simulink model "v00_0A_0E"  (R2022b)
settings: Solver=FixedStepDiscrete  StartTime=0.0  StopTime=8000  FixedStep=SampleTime  MaxStep=Contactors_StepTime_msec  RelTol=1e-3  EnableMultiTasking=on
undefined symbols (not defined in the file): A_to_mA, BalancingTempGroup, canChannel, CapacityFactor, CC_Inputs, CellSOC, ChargeState, ContactorsFlags, DiscIntNeverNeededParam, gEN_Contactors_StepTime_msec, Ion, isDynamicCurrentEn, Lithium, maxAllowedImbalance, nCells_parallel, nCells_series, nCellTempGrps, PermanentFailRecoveryTrigger, ProtectionFlags, RBal_ohm, SampleTime, sigbuilder_block, StLineEq_varA, StLineEq_varB, TempSelectForDCL, Thresholds, V_to_mV
libraries: simulink x32, spsIdealSwitchLib x21, spsBatteryLib x20, spsSeriesRLCBranchLib x20, spsVoltageMeasurementLib x20, canmsglib x4, canlib x3, dspstat3 x2, spspowerguiLib x2, spsControlledCurrentSourceLib x1, spsCurrentMeasurementLib x1
(part 3 of 7)

== system v00_0A_0E/CellBalancing ==
  note: BalanceEn_atRest is added in Input Processing block for offline cell balancing
  note: BalanceEn = 1 is added in statemachine when transitioning from Lobby to even balancing
  BalancingTempGroup : Inport
  maxAllowedImbalance : Inport  Port=2
  StLineEq_varA : Inport  Port=3
  StLineEq_varB : Inport  Port=4
  Thresholds : Inport  Port=5
  DataPipeline : Inport  Port=6
  BalancingStateMachine : Stateflow chart  TreatAsAtomicUnit=on
      settings: PortSchema="{\"entries\":[{\"content\":{\"sides\":[{\"content\":{\"connectorIds\":[\"In1\",\"In3\",\"In2\",\"In4\",\"In6\",\"In5\"]},\"type\":\"ConnectorPlacement.EquallySpacedRectSide\",\"uuid\":\"2851f266-9e46-4eaf-8471-39569b09250f\"},{\"content\":{\"connectorIds\":[\"Out2\",\"Out1\"],\"side\":\"RIGHT\"},\"type\":\"ConnectorPlacement.EquallySpacedRectSide\",\"uuid\":\"62b89b69-68b5-43db-8812-bb8e11eec61f\"},{\"content\":{\"connectorIds\":[],\"side\":\"TOP\"},\"type\":\"ConnectorPlacement.EquallySpacedRectSide\",\"uuid\":\"40469b38-8e93-4311-b6ae-b85f5792b8b2\"},{\"content\":{\"connectorIds\":[],\"side\":\"BOTTOM\"},\"type\":\"ConnectorPlacement.EquallySpacedRectSide\",\"uuid\":\"8aed0a4d-23dc-44c4-b683-dda48b400f95\"}]},\"type\":\"ConnectorPlacement.EquallySpacedConnector\",\"uuid\":\"3b02c2cb-c692-4407-a922-660092207305\"}],\"packageUris\":[\"http://schema.mathworks.com/mf0/Connector/R2020b\"],\"version\":\"1.0\"}"
  Bus Creator : BusCreator  Inputs=3  OutDataTypeStr=Bus: CellBalancingOutputBus  NonVirtualBus=on
  Bus Selector1 : BusSelector  OutputSignals=VoltageSenseBus.mV_max,nCells_series,VoltageSenseBus.Voltages_mV,VoltageSenseBus.mV_min
  InputProcessing : Subsystem
  Subtract : Sum  Inputs=+-  AccumDataTypeStr=int32
  BalanceCmd : Outport
  CellBalancingOutput : Outport  Port=2
  wires:
  InputProcessing/1(BalanceEn) -> BalancingStateMachine/4(BalanceEn), Bus Creator/2  "BalanceEn"
  BalancingStateMachine/1(BalanceCmd) -> BalanceCmd/1  "BalanceCmd"
  DataPipeline/1 -> InputProcessing/1(DataPipeline), Bus Selector1/1  "DataPipeline"
  Thresholds/1 -> InputProcessing/6(Thresholds), BalancingStateMachine/5(Thresholds)  "Thresholds"
  Bus Creator/1 -> CellBalancingOutput/1  "CellBalancingOutput"
  StLineEq_varA/1 -> InputProcessing/3(StLineEq_varA)  "StLineEq_varA"
  StLineEq_varB/1 -> InputProcessing/4(StLineEq_varB)  "StLineEq_varB"
  BalancingTempGroup/1 -> InputProcessing/5(BalancingTempGroup)  "BalancingTempGroup"
  InputProcessing/2(BalancingTimeOn_msec) -> BalancingStateMachine/6(BalancingTimeOn_msec)  "BalancingTimeOn_msec"
  Bus Selector1/2 -> BalancingStateMachine/1(nCells_series)  "<nCells_series>"
  Bus Selector1/3 -> BalancingStateMachine/3(Voltage_mV)  "<Voltages_mV>"
  Subtract/1 -> Bus Creator/1  "MaxImbalance_mV"
  BalancingStateMachine/2(CurrentBalancingState) -> Bus Creator/3  "CurrentBalancingState"
  Bus Selector1/4 -> Subtract/2, BalancingStateMachine/2(mV_min)  "<mV_min>"
  Bus Selector1/1 -> Subtract/1  "<mV_max>"
  maxAllowedImbalance/1 -> InputProcessing/2(MaxAllowedImbalance)

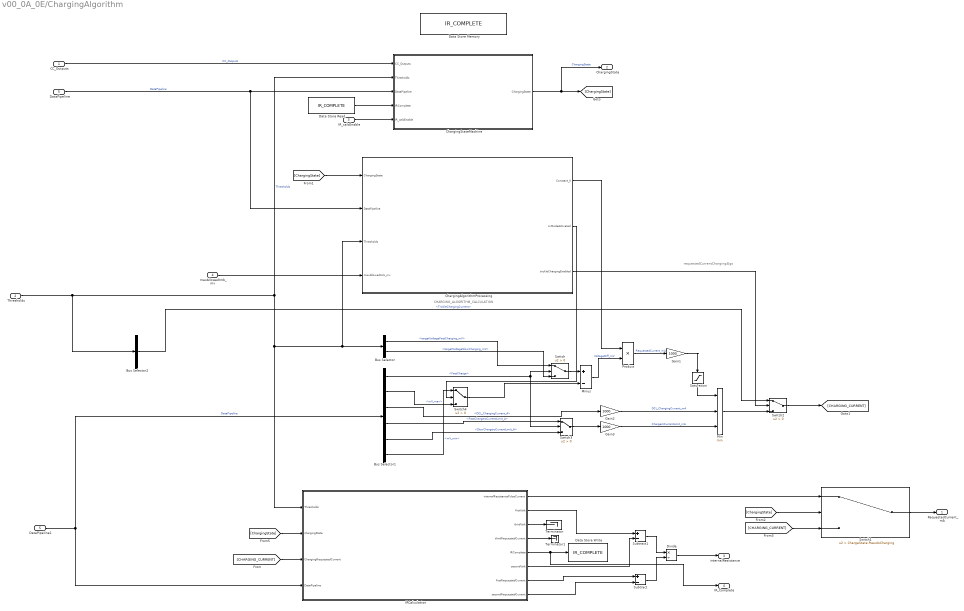
== system v00_0A_0E/ChargingAlgorithm ==
  note: requestedCurrentChargingAlgo
  note: CHARGING_ALGORITHM_CALCULATION
  CC_Outputs : Inport
  Thresholds : Inport  Port=2
  IR_calcEnable : Inport  Port=3
  maxAllowedImb_mv : Inport  Port=4
  DataPipeline : Inport  Port=5
  Bus Selector : BusSelector  OutputSignals=targetVoltageFastCharging_mV,targetVoltageSlowCharging_mV
  Bus Selector1 : BusSelector  OutputSignals=VCU.FastCharge,VoltageSenseBus.mV_max,DCL_ChargingCurrent_A,VCU.FastChargersCurrentLimit_A,VCU.SlowChargersCurrentLimit_A,VoltageSenseBus.mV_min
  Bus Selector2 : BusSelector  OutputSignals=TrickleChargingCurrent
  ChargingAlgorithmProcessing : Stateflow chart  TreatAsAtomicUnit=on
  ChargingStateMachine : Stateflow chart  TreatAsAtomicUnit=on
  Data Store Memory : DataStoreMemory  DataStoreName=IR_COMPLETE  WriteAfterWriteMsg=warning  ShowAdditionalParam=off  OutDataTypeStr=boolean
  Data Store Read : DataStoreRead  DataStoreName=IR_COMPLETE  IndexOptions=Index vector (dialog)  Indices=1  OutputSizes=1
  Data Store Write : DataStoreWrite  DataStoreName=IR_COMPLETE  IndexOptions=Index vector (dialog)  Indices=1  OutputSizes=1
  DataPipeline1 : InportShadow  Port=5
  Divide : Product  Inputs=*/  OutDataTypeStr=double
  Gain1 : Gain  Gain=1000
  Gain2 : Gain  Gain=1000
  Gain3 : Gain  Gain=1000
  IRCalculation : Stateflow chart  TreatAsAtomicUnit=on
      settings: PortSchema="{\"entries\":[{\"content\":{\"sides\":[{\"content\":{\"connectorIds\":[\"In3\",\"In2\",\"In4\",\"In1\"]},\"type\":\"ConnectorPlacement.EquallySpacedRectSide\",\"uuid\":\"09f3344b-a7a5-4c58-b859-bc86e5255ecc\"},{\"content\":{\"connectorIds\":[\"Out1\",\"Out5\",\"Out6\",\"Out7\",\"Out8\",\"Out4\",\"Out3\",\"Out2\"],\"side\":\"RIGHT\"},\"type\":\"ConnectorPlacement.EquallySpacedRectSide\",\"uuid\":\"d87cb124-6959-4bc9-a690-eca1c3acb93d\"},{\"content\":{\"connectorIds\":[],\"side\":\"TOP\"},\"type\":\"ConnectorPlacement.EquallySpacedRectSide\",\"uuid\":\"d4f2166d-1afb-4cd8-92f5-d7d1af5b4065\"}]},\"type\":\"ConnectorPlacement.EquallySpacedConnector\",\"uuid\":\"753fa2af-6988-4d89-a789-6b550e8286be\"}],\"packageUris\":[\"http://schema.mathworks.com/mf0/Connector/R2020b\"],\"version\":\"1.0\"}"
  Min : MinMax  Inputs=3
  Minus : Sum  Inputs=+-  OutDataTypeStr=int32
  Product : Product  OutDataTypeStr=int32
  Saturation : Saturate  UpperLimit=200000  LowerLimit=0
  Subtract : Sum  Inputs=+-
  Subtract1 : Sum  Inputs=+-
  Switch{,2..4} (4 alike) : Switch  Criteria=u2 > Threshold  SaturateOnIntegerOverflow=off  InputSameDT=off
  Switch1 : Switch  Criteria=u2 > Threshold  Threshold=ChargeState.PseudoCharging  SaturateOnIntegerOverflow=off  InputSameDT=off
  Terminator : Terminator
  Terminator1 : Terminator
  RequestedCurrent_mA : Outport
  ChargingState : Outport  Port=2
  internalResistance : Outport  Port=3
  IR_Complete : Outport  Port=4
  wires:
  IRCalculation/7(thirdRequestedCurrent) -> Terminator1/1
  IRCalculation/1(internalResistancePulseCurrent) -> Switch1/1
  Subtract/1 -> Divide/2
  IRCalculation/2(secondRequestedCurrent) -> Subtract/2
  IRCalculation/4(secondVolt) -> Subtract1/2
  IRCalculation/3(firstRequestedCurrent) -> Subtract/1
  IRCalculation/5(firstVolt) -> Subtract1/1
  Subtract1/1 -> Divide/1
  CC_Outputs/1 -> ChargingStateMachine/1(CC_Outputs)  "CC_Outputs"
  [ChargingState] -> ChargingAlgorithmProcessing/1(ChargingState)
  IRCalculation/6(thirdVolt) -> Terminator/1
  Bus Selector1/6 -> Switch4/1  "<mV_min>"
  Bus Selector2/1 -> Switch2/1  "<TrickleChargingCurrent>"
  Bus Selector1/3 -> Gain2/1  "<DCL_ChargingCurrent_A>"
  Gain3/1 -> Min/3  "ChargersCurrentLimit_mA"
  Bus Selector1/1 -> Switch3/2, Switch/2  "<FastCharge>"
  Switch3/1 -> Gain3/1
  Gain2/1 -> Min/2  "DCL_ChargingCurrent_mA"
  Minus/1 -> Product/2  "VoltageDiff_mV"
  ChargingAlgorithmProcessing/3(trickleChargingEnabled) -> Switch2/2
  Min/1 -> Switch2/3
  DataPipeline/1 -> ChargingAlgorithmProcessing/2(DataPipeline), ChargingStateMachine/3(DataPipeline)  "DataPipeline"
  Switch/1 -> Minus/1
  ChargingAlgorithmProcessing/1(Constant_K) -> Product/1
  DataPipeline1/1 -> Bus Selector1/1, IRCalculation/1(DataPipeline)  "DataPipeline"
  Product/1 -> Gain1/1  "RequestedCurrent_mA"
  Bus Selector1/5 -> Switch3/3  "<SlowChargersCurrentLimit_A>"
  ChargingAlgorithmProcessing/2(cvModeActivated) -> Switch4/2
  Bus Selector/2 -> Switch/3  "<targetVoltageSlowCharging_mV>"
  Thresholds/1 -> Bus Selector2/1, ChargingStateMachine/2(Thresholds), Bus Selector/1, ChargingAlgorithmProcessing/3(Thresholds), IRCalculation/3(Thresholds)  "Thresholds"
  Bus Selector1/4 -> Switch3/1  "<FastChargersCurrentLimit_A>"
  Bus Selector/1 -> Switch/1  "<targetVoltageFastCharging_mV>"
  Gain1/1 -> Saturation/1
  Switch4/1 -> Minus/2
  IR_calcEnable/1 -> ChargingStateMachine/5(IR_calcEnable)
  maxAllowedImb_mv/1 -> ChargingAlgorithmProcessing/4(maxAllowedImb_mv)
  Saturation/1 -> Min/1
  Bus Selector1/2 -> Switch4/3  "<mV_max>"
  [ChargingState] -> Switch1/2
  Switch1/1 -> RequestedCurrent_mA/1
  Switch2/1 -> [CHARGING_CURRENT]
  [CHARGING_CURRENT] -> IRCalculation/4(ChargingRequestedCurrent)
  [CHARGING_CURRENT] -> Switch1/3
  Divide/1 -> internalResistance/1
  IRCalculation/8(IRComplete) -> IR_Complete/1, Data Store Write/1
  Data Store Read/1 -> ChargingStateMachine/4(IRComplete)
  ChargingStateMachine/1(ChargingState) -> ChargingState/1, [ChargingState]  "ChargingState"
  [ChargingState] -> IRCalculation/2(chargingState)

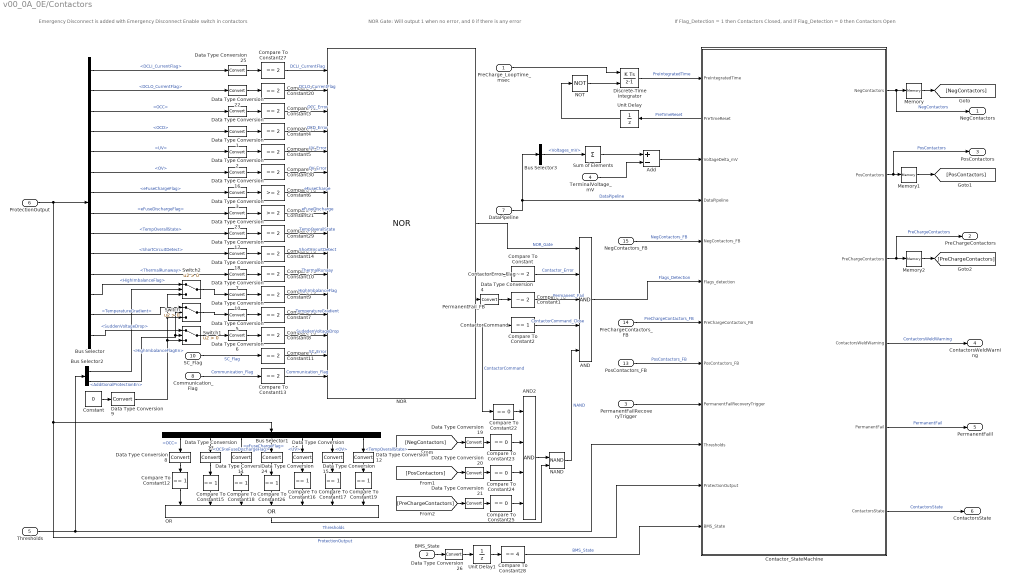
== system v00_0A_0E/Contactors ==
  note: Emergency Disconnect is added with Emergency Disconnect Enable switch in contactors
  note: If Flag_Detection = 1 then Contactors Closed, and if Flag_Detection = 0 then Contactors Open
  note: NOR Gate: Will output 1 when no error, and 0 if there is any error
  PreCharge_LoopTime_msec : Inport
  BMS_State : Inport  Port=2
  PermanentFailRecoveryTrigger : Inport  Port=3
  TerminalVoltage_mV : Inport  Port=4
  Thresholds : Inport  Port=5
  ProtectionOutput : Inport  Port=6
  DataPipeline : Inport  Port=7
  Communication_Flag : Inport  Port=8
  ContactorCommand : Inport  Port=9
  SC_Flag : Inport  Port=10
  PermanentFail_FB : Inport  Port=11
  ContactorError_Flag : Inport  Port=12
  PosContactors_FB : Inport  Port=13
  PreChargeContactors_FB : Inport  Port=14
  NegContactors_FB : Inport  Port=15
  AND : Logic  Inputs=5  IconShape=distinctive  AllPortsSameDT=off  OutDataTypeStr=boolean
  AND2 : Logic  Inputs=4  IconShape=distinctive  AllPortsSameDT=off  OutDataTypeStr=boolean
  Add : Sum  Inputs=+-
  Bus Selector : BusSelector  OutputSignals=DCLI_CurrentFlag,DCLO_CurrentFlag,OCC,OCD,UV,OV,eFuseChargeFlag,eFuseDischargeFlag,TempOverallState,ShortCircuitDetect,ThermalRunaway,HighImbalanceFlag,TemperatureGradient,SuddenVoltageDrop
  Bus Selector1 : BusSelector  OutputSignals=OCC,OCD,eFuseChargeFlag,eFuseDischargeFlag,UV,OV,TempOverallState
  Bus Selector2 : BusSelector  OutputSignals=HighImbalanceFlagEn,AdditionalProtectionEn
  Bus Selector3 : BusSelector  OutputSignals=VoltageSenseBus.Voltages_mV
  Compare To Constant : simulink/Logic and Bit Operations/Compare To Constant  relop=~=  const=2  OutDataTypeStr=boolean
  Compare To Constant1 : simulink/Logic and Bit Operations/Compare To Constant  relop=~=  const=2  OutDataTypeStr=boolean
  Compare To Constant{3..5,7..11,13..14,20,27,29..30} (14 alike) : simulink/Logic and Bit Operations/Compare To Constant  relop===  const=2  OutDataTypeStr=boolean
  Compare To Constant{2,12,15..19,26} (8 alike) : simulink/Logic and Bit Operations/Compare To Constant  relop===  const=1  OutDataTypeStr=boolean
  Compare To Constant21 : simulink/Logic and Bit Operations/Compare To Constant  relop=>=  const=2  OutDataTypeStr=boolean
  Compare To Constant{22..25} (4 alike) : simulink/Logic and Bit Operations/Compare To Constant  relop===  const=0  OutDataTypeStr=boolean
  Compare To Constant28 : simulink/Logic and Bit Operations/Compare To Constant  relop===  const=4  OutDataTypeStr=boolean
  Compare To Constant6 : simulink/Logic and Bit Operations/Compare To Constant  relop=>=  const=2  OutDataTypeStr=boolean
  Constant : Constant  Value=0  OutDataTypeStr=uint8
  Contactor_StateMachine : Stateflow chart  TreatAsAtomicUnit=on
      settings: PortSchema="{\"entries\":[{\"content\":{\"sides\":[{\"content\":{\"connectorIds\":[\"In1\",\"Out1\",\"In2\",\"In5\",\"In6\",\"In3\",\"In7\",\"In8\",\"In9\",\"In4\",\"In10\",\"In11\"]},\"type\":\"ConnectorPlacement.EquallySpacedRectSide\",\"uuid\":\"585ccc14-d5fb-43f7-bbc3-e9debde63d5b\"},{\"content\":{\"connectorIds\":[\"Out2\",\"Out3\",\"Out4\",\"Out5\",\"Out6\",\"Out7\"],\"side\":\"RIGHT\"},\"type\":\"ConnectorPlacement.EquallySpacedRectSide\",\"uuid\":\"9f335c67-e84f-4d2b-8ce3-ad147bd210d5\"},{\"content\":{\"connectorIds\":[],\"side\":\"TOP\"},\"type\":\"ConnectorPlacement.EquallySpacedRectSide\",\"uuid\":\"58b4bb50-48c3-4ece-b5a6-da56bbf5650f\"}]},\"type\":\"ConnectorPlacement.EquallySpacedConnector\",\"uuid\":\"a721c968-75ef-472f-94e6-7730f73173d4\"}],\"packageUris\":[\"http://schema.mathworks.com/mf0/Connector/R2020b\"],\"version\":\"1.0\"}"
  Data Type Conversion{,1..26} (27 alike) : DataTypeConversion  SaturateOnIntegerOverflow=off  RndMeth=Floor
  Discrete-Time Integrator : DiscreteIntegrator  gainval=1  ExternalReset=level  SampleTime=-1  ICPrevOutput=DiscIntNeverNeededParam  ICPrevScaledInput=DiscIntNeverNeededParam
  Memory : Memory  InitialCondition=ContactorsFlags.Open  InheritSampleTime=on
  Memory1 : Memory  InitialCondition=ContactorsFlags.Open  InheritSampleTime=on
  Memory2 : Memory  InitialCondition=ContactorsFlags.Open  InheritSampleTime=on
  NAND : Logic  Operator=NAND  IconShape=distinctive  AllPortsSameDT=off  OutDataTypeStr=boolean
  NOR : Logic  Operator=NOR  Inputs=16  IconShape=distinctive  AllPortsSameDT=off  OutDataTypeStr=boolean
  NOT : Logic  Operator=NOT  IconShape=distinctive  AllPortsSameDT=off  OutDataTypeStr=boolean
  OR : Logic  Operator=OR  Inputs=7  IconShape=distinctive  AllPortsSameDT=off  OutDataTypeStr=boolean
  Sum of Elements : Sum  Inputs=+
  Switch : Switch  Criteria=u2 > Threshold  SaturateOnIntegerOverflow=off  InputSameDT=off
  Switch1 : Switch  Criteria=u2 > Threshold  SaturateOnIntegerOverflow=off  InputSameDT=off
  Switch2 : Switch  Criteria=u2 > Threshold  SaturateOnIntegerOverflow=off  InputSameDT=off
  Unit Delay : UnitDelay  SampleTime=-1  HasFrameUpgradeWarning=on
  Unit Delay1 : UnitDelay  SampleTime=-1  HasFrameUpgradeWarning=on
  NegContactors : Outport
  PreChargeContactors : Outport  Port=2
  PosContactors : Outport  Port=3
  ContactorsWeldWarning : Outport  Port=4
  PermanentFaiil : Outport  Port=5
  ContactorsState : Outport  Port=6
  wires:
  NOR/1 -> AND/1  "NOR_Gate"
  ContactorError_Flag/1 -> Compare To Constant/1
  Compare To Constant1/1 -> AND/3  "Permanent_Fail"
  Compare To Constant/1 -> AND/2  "Contactor_Error"
  Compare To Constant2/1 -> AND/4  "ContactorCommand_Close"
  PermanentFail_FB/1 -> Data Type Conversion4/1
  SC_Flag/1 -> Compare To Constant11/1  "SC_Flag"
  ContactorCommand/1 -> Compare To Constant22/1, Compare To Constant2/1  "ContactorCommand"
  Communication_Flag/1 -> Compare To Constant13/1  "Communication_Flag"
  AND/1 -> Contactor_StateMachine/3(Flags_detection)  "Flags_Detection"
  NegContactors_FB/1 -> Contactor_StateMachine/6(NegContactors_FB)  "NegContactors_FB"
  PreChargeContactors_FB/1 -> Contactor_StateMachine/7(PreChargeContactors_FB)  "PreChargeContactors_FB"
  PosContactors_FB/1 -> Contactor_StateMachine/8(PosContactors_FB)  "PosContactors_FB"
  ProtectionOutput/1 -> Bus Selector1/1, Contactor_StateMachine/10(ProtectionOutput), Bus Selector/1  "ProtectionOutput"
  Bus Selector1/1 -> Data Type Conversion8/1  "<OCC>"
  Compare To Constant22/1 -> AND2/1
  AND2/1 -> NAND/1
  NAND/1 -> AND/5  "NAND"
  OR/1 -> NAND/2
  Compare To Constant23/1 -> AND2/2
  Compare To Constant24/1 -> AND2/3
  Compare To Constant25/1 -> AND2/4
  [NegContactors] -> Data Type Conversion19/1
  [PosContactors] -> Data Type Conversion20/1
  [PreChargeContactors] -> Data Type Conversion21/1
  Contactor_StateMachine/3(PosContactors) -> PosContactors/1, Memory1/1  "PosContactors"
  Contactor_StateMachine/4(PreChargeContactors) -> PreChargeContactors/1, Memory2/1  "PreChargeContactors"
  Thresholds/1 -> Contactor_StateMachine/4(Thresholds), Bus Selector2/1  "Thresholds"
  Contactor_StateMachine/2(NegContactors) -> NegContactors/1, Memory/1  "NegContactors"
  DataPipeline/1 -> Bus Selector3/1, Contactor_StateMachine/5(DataPipeline)  "DataPipeline"
  Data Type Conversion/1 -> Compare To Constant3/1
  Data Type Conversion1/1 -> Compare To Constant4/1
  Data Type Conversion2/1 -> Compare To Constant5/1
  Data Type Conversion3/1 -> Compare To Constant6/1
  Data Type Conversion7/1 -> Compare To Constant10/1
  Data Type Conversion8/1 -> Compare To Constant12/1
  Bus Selector1/7 -> Data Type Conversion12/1  "<TempOverallState>"
  Bus Selector1/2 -> Data Type Conversion13/1  "<OCD>"
  Data Type Conversion13/1 -> Compare To Constant15/1
  Bus Selector1/5 -> Data Type Conversion14/1  "<UV>"
  Data Type Conversion14/1 -> Compare To Constant16/1
  Bus Selector1/6 -> Data Type Conversion15/1  "<OV>"
  Data Type Conversion15/1 -> Compare To Constant17/1
  Data Type Conversion16/1 -> Compare To Constant30/1
  Data Type Conversion17/1 -> Compare To Constant29/1
  Data Type Conversion18/1 -> Compare To Constant14/1
  Data Type Conversion19/1 -> Compare To Constant23/1
  Data Type Conversion20/1 -> Compare To Constant24/1
  Data Type Conversion21/1 -> Compare To Constant25/1
  Memory/1 -> [NegContactors]
  Memory1/1 -> [PosContactors]
  Memory2/1 -> [PreChargeContactors]
  Contactor_StateMachine/5(ContactorsWeldWarning) -> ContactorsWeldWarning/1  "ContactorsWeldWarning"
  Data Type Conversion4/1 -> Compare To Constant1/1
  Data Type Conversion5/1 -> Compare To Constant7/1
  Contactor_StateMachine/6(PermanentFail) -> PermanentFaiil/1  "PermanentFail"
  PermanentFailRecoveryTrigger/1 -> Contactor_StateMachine/9(PermanentFailRecoveryTrigger)
  Data Type Conversion6/1 -> Compare To Constant8/1
  Contactor_StateMachine/7(ContactorsState) -> ContactorsState/1  "ContactorsState"
  Switch/1 -> Data Type Conversion5/1
  Switch1/1 -> Data Type Conversion6/1
  Constant/1 -> Data Type Conversion9/1
  Bus Selector2/2 -> Switch/2, Switch1/2  "<AdditionalProtectionEn>"
  Data Type Conversion9/1 -> Switch1/3, Switch2/3, Switch/3
  Switch2/1 -> Data Type Conversion10/1
  Data Type Conversion10/1 -> Compare To Constant9/1
  Compare To Constant3/1 -> NOR/3  "OCC_Error"
  Compare To Constant4/1 -> NOR/4  "OCD_Error"
  Compare To Constant5/1 -> NOR/5  "UV_Error"
  Bus Selector/4 -> Data Type Conversion1/1  "<OCD>"
  Bus Selector/3 -> Data Type Conversion/1  "<OCC>"
  Bus Selector/6 -> Data Type Conversion16/1  "<OV>"
  Bus Selector/9 -> Data Type Conversion17/1  "<TempOverallState>"
  Bus Selector/10 -> Data Type Conversion18/1  "<ShortCircuitDetect>"
  Bus Selector/11 -> Data Type Conversion7/1  "<ThermalRunaway>"
  Bus Selector/12 -> Switch2/1  "<HighImbalanceFlag>"
  Bus Selector/13 -> Switch/1  "<TemperatureGradient>"
  Bus Selector/14 -> Switch1/1  "<SuddenVoltageDrop>"
  Data Type Conversion12/1 -> Compare To Constant19/1
  Data Type Conversion11/1 -> Compare To Constant18/1
  Bus Selector1/3 -> Data Type Conversion11/1  "<eFuseChargeFlag>"
  Bus Selector2/1 -> Switch2/2  "<HighImbalanceFlagEn>"
  Bus Selector/5 -> Data Type Conversion2/1  "<UV>"
  Compare To Constant13/1 -> NOR/16  "Communication_Flag"
  Compare To Constant11/1 -> NOR/15  "SC_Error"
  Compare To Constant8/1 -> NOR/14  "SudedenVoltageDrop"
  Compare To Constant7/1 -> NOR/13  "TemperatureGradient"
  Compare To Constant9/1 -> NOR/12  "HighImbalanceFlag"
  Compare To Constant10/1 -> NOR/11  "ThermalRunaay"
  Compare To Constant14/1 -> NOR/10  "ShortCircuitDetect"
  Compare To Constant29/1 -> NOR/9  "TempOverallState"
  Compare To Constant30/1 -> NOR/6  "OV_Error"
  Compare To Constant6/1 -> NOR/7  "eFuseCharge"
  Bus Selector/7 -> Data Type Conversion3/1  "<eFuseChargeFlag>"
  Data Type Conversion23/1 -> Compare To Constant21/1
  Bus Selector/8 -> Data Type Conversion23/1  "<eFuseDischargeFlag>"
  Compare To Constant21/1 -> NOR/8  "eFuseDischarge"
  Compare To Constant12/1 -> OR/1
  Compare To Constant15/1 -> OR/2
  Compare To Constant18/1 -> OR/3
  Compare To Constant19/1 -> OR/7
  Compare To Constant17/1 -> OR/6
  Compare To Constant16/1 -> OR/5
  Data Type Conversion24/1 -> Compare To Constant26/1
  Bus Selector1/4 -> Data Type Conversion24/1  "<eFuseDischargeFlag>"
  Compare To Constant26/1 -> OR/4
  Bus Selector3/1 -> Sum of Elements/1  "<Voltages_mV>"
  TerminalVoltage_mV/1 -> Add/2
  Sum of Elements/1 -> Add/1
  Add/1 -> Contactor_StateMachine/2(VoltageDelta_mV)
  Data Type Conversion22/1 -> Compare To Constant20/1
  Data Type Conversion25/1 -> Compare To Constant27/1
  Bus Selector/1 -> Data Type Conversion25/1  "<DCLI_CurrentFlag>"
  Bus Selector/2 -> Data Type Conversion22/1  "<DCLO_CurrentFlag>"
  Compare To Constant27/1 -> NOR/1  "DCLI_CurrentFlag"
  Compare To Constant20/1 -> NOR/2  "DCLO_CurrentFlag"
  NOT/1 -> Discrete-Time Integrator/2
  Unit Delay/1 -> NOT/1
  Contactor_StateMachine/1(PreTimeReset) -> Unit Delay/1  "PreTimeReset"
  PreCharge_LoopTime_msec/1 -> Discrete-Time Integrator/1
  Discrete-Time Integrator/1 -> Contactor_StateMachine/1(PreIntegratedTime)  "PreIntegratedTime"
  Compare To Constant28/1 -> Contactor_StateMachine/11(BMS_State)  "BMS_State"
  Data Type Conversion26/1 -> Unit Delay1/1
  BMS_State/1 -> Data Type Conversion26/1
  Unit Delay1/1 -> Compare To Constant28/1

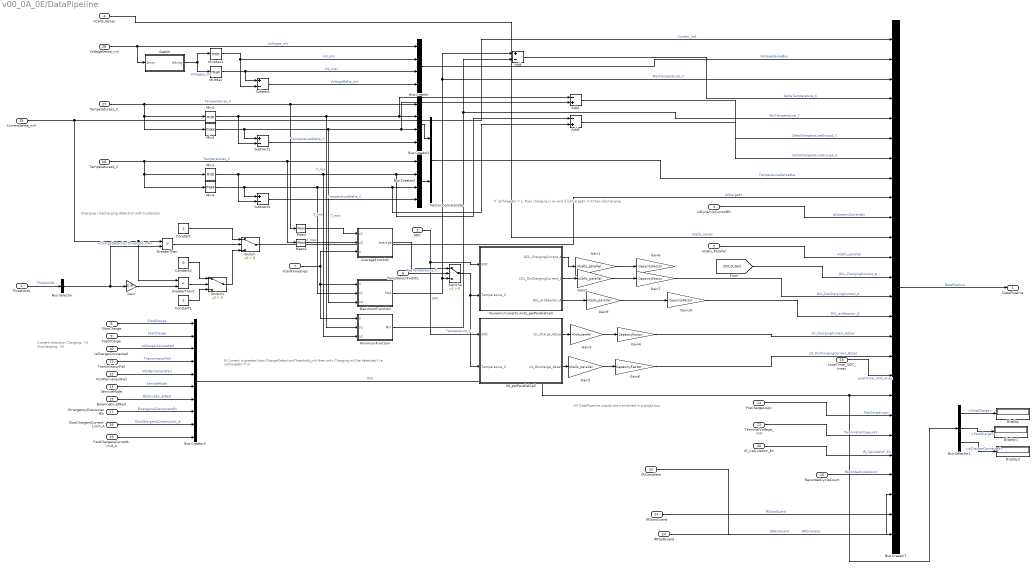
== system v00_0A_0E/DataPipeline ==
  note: All DataPipeline ouputs are combined in a single bus
  note: If Current is greater than ChargeDetectionThreshold_mA then only Charging will be detected (i.e. isChargeEn = 1)
  note: If isChargeEn = 1, then charging is on and if isChargeEn = 0 then discharging
  note: Charging / discharging detection with hysteresis
  note: Current direction
      | Charging: >0
      | Discharging: <0
  Thresholds : Inport
  SOC : Inport  Port=2
  isDynamicCurrentEn : Inport  Port=3
  nCells_Series : Inport  Port=4
  nCells_Parallel : Inport  Port=5
  TempSelectForDCL : Inport  Port=6
  nCellTempGrps : Inport  Port=7
  SlowCharge : Inport  Port=8
  FastCharge : Inport  Port=9
  isChargerConnected : Inport  Port=10
  TransmissionFail : Inport  Port=11
  VCUPermanentFail : Inport  Port=12
  ServiceMode : Inport  Port=13
  PreChargeLogic : Inport  Port=14
  BalanceEn_atRest : Inport  Port=15
  LoopTimer_SOC_msec : Inport  Port=16
  EmergencyDisconnectEn : Inport  Port=17
  SlowChargersCurrentLimit_A : Inport  Port=18
  FastChargersCurrentLimit_A : Inport  Port=19
  IR_Calculation_En : Inport  Port=20
  TerminalVoltage_mV : Inport  Port=21
  IRComplete : Inport  Port=22
  IRSlowGuard : Inport  Port=23
  IRFastGuard : Inport  Port=24
  RecordedCycleCount : Inport  Port=25  OutDataTypeStr=uint32
  Temperatures2_C : Inport  Port=26
  Temperatures1_C : Inport  Port=27
  VoltageSense_mV : Inport  Port=28
  CurrentSense_mA : Inport  Port=29
  Add : Sum  Inputs=+-  OutDataTypeStr=int16
  Add1 : Sum  Inputs=-+  OutDataTypeStr=int16
  Add2 : Sum  Inputs=-+  OutDataTypeStr=int16
  AverageFunction : MATLAB Function  TreatAsAtomicUnit=on
      settings: RTWFcnNameOpts=Use subsystem name  RTWFileNameOpts=Use subsystem name
  Bus Creator : BusCreator  Inputs=4  OutDataTypeStr=Bus: VoltageSenseBus  NonVirtualBus=on
  Bus Creator1 : BusCreator  Inputs=4  OutDataTypeStr=Bus: TemperatureSenseBus  NonVirtualBus=on
  Bus Creator2 : BusCreator  Inputs=4  OutDataTypeStr=Bus: TemperatureSenseBus  NonVirtualBus=on
  Bus Creator3 : BusCreator  Inputs=10  OutDataTypeStr=Bus: VCU  NonVirtualBus=on
  Bus Creator7 : BusCreator  Inputs=26  OutDataTypeStr=Bus: DataPipelineBus  NonVirtualBus=on
  Bus Selector : BusSelector  OutputSignals=ChargeDetectionThreshold_mA
  Bus Selector1 : BusSelector  OutputSignals=SlowCharge,FastCharge,isChargerConnected
  Constant : Constant  OutDataTypeStr=uint8
  Constant1 : Constant  OutDataTypeStr=uint8
  Constant2 : Constant  Value=0  OutDataTypeStr=uint8
  Display : Display
  Display1 : Display
  Display2 : Display
  DynamicCurrentLimits_perParallelCell : MATLAB Function  TreatAsAtomicUnit=on
      settings: RTWFcnNameOpts=Use subsystem name  RTWFileNameOpts=Use subsystem name
  Gain : Gain  Gain=0.9
  Gain{1..3,5,9} (5 alike) : Gain  Gain=nCells_parallel
  Gain10 : Gain  Gain=CapacityFactor  OutDataTypeStr=single
  Gain4 : Gain  Gain=CapacityFactor  ParamDataTypeStr=single  OutDataTypeStr=single
  Gain6 : Gain  Gain=CapacityFactor  OutDataTypeStr=single
  Gain7 : Gain  Gain=CapacityFactor  OutDataTypeStr=single
  Gain8 : Gain  Gain=CapacityFactor  ParamDataTypeStr=single  OutDataTypeStr=single
  GetN3 : Subsystem
  GreaterThan : RelationalOperator  Operator=>  OutDataTypeStr=boolean  RndMeth=Simplest  InputSameDT=off
  GreaterThan1 : RelationalOperator  Operator=<  OutDataTypeStr=boolean  RndMeth=Simplest  InputSameDT=off
  I2t_perParallelCell : MATLAB Function  TreatAsAtomicUnit=on
      settings: RTWFcnNameOpts=Use subsystem name  RTWFileNameOpts=Use subsystem name
  MaximumFunction : MATLAB Function  TreatAsAtomicUnit=on
      settings: RTWFcnNameOpts=Use subsystem name  RTWFileNameOpts=Use subsystem name
  Mean : dspstat3/Mean  run=off  InputProcessing=Columns as channels (frame based)  reset_popup=None  directionMode=Each column  dimension=1  roiEnable=off  roiType=Rectangles  roiPortion=Entire ROI  roiOutput=Individual statistics for each ROI  roiFlag=off  roundingMode=Floor  overflowMode=off  outputDataTypeStr=Inherit: Same as accumulator  outputMin=[]  outputMax=[]  outputLastDataTypeStr=Inherit: Same as accumulator
  Mean1 : dspstat3/Mean  run=off  InputProcessing=Columns as channels (frame based)  reset_popup=None  directionMode=Each column  dimension=1  roiEnable=off  roiType=Rectangles  roiPortion=Entire ROI  roiOutput=Individual statistics for each ROI  roiFlag=off  roundingMode=Floor  overflowMode=off  outputDataTypeStr=Inherit: Same as accumulator  outputMin=[]  outputMax=[]  outputLastDataTypeStr=Inherit: Same as accumulator
  Min1 : MinMax  OutDataTypeStr=int16
  Min2 : MinMax  OutDataTypeStr=int16
  Min3 : MinMax  Function=max  OutDataTypeStr=int16
  Min4 : MinMax  Function=max  OutDataTypeStr=int16
  MinMax : MinMax  Function=max
  MinMax2 : MinMax  InputSameDT=on
  MinimumFunction : MATLAB Function  TreatAsAtomicUnit=on
      settings: RTWFcnNameOpts=Use subsystem name  RTWFileNameOpts=Use subsystem name
  Subtract : Sum  Inputs=+-
  Subtract1 : Sum  Inputs=+-  OutDataTypeStr=int16
  Subtract2 : Sum  Inputs=+-  OutDataTypeStr=int16
  Switch : Switch  Criteria=u2 > Threshold  OutDataTypeStr=uint8  SaturateOnIntegerOverflow=off  InputSameDT=off
  Switch1 : Switch  Criteria=u2 > Threshold  OutDataTypeStr=int32  SaturateOnIntegerOverflow=off  InputSameDT=off
  Switch4 : Switch  Criteria=u2 > Threshold  SaturateOnIntegerOverflow=off  InputSameDT=off
  Vector Concatenate : Concatenate
  DataPipeline : Outport
  wires:
  MinMax/1 -> Subtract/1, Bus Creator/3  "mV_max"
  Min3/1 -> Subtract1/1, MaximumFunction/3(u2), Bus Creator1/3, Add1/2  "T_max"
  Min2/1 -> Subtract1/2, MinimumFunction/2(u1), Bus Creator1/2, Add1/1  "T_min"
  Subtract/1 -> Bus Creator/4  "VoltageDelta_mV"
  Subtract1/1 -> Bus Creator1/4  "TemperatureDelta_C"
  CurrentSense_mA/1 -> GreaterThan/1, GreaterThan1/1, Bus Creator7/1  "Current_mA"
  VoltageSense_mV/1 -> GetN3/1(Array), Bus Creator/1  "Voltages_mV"
  Constant/1 -> Switch/1
  GreaterThan/1 -> Switch/2
  Switch1/1 -> Switch/3
  GreaterThan1/1 -> Switch1/2
  Constant1/1 -> Switch1/3
  Gain/1 -> GreaterThan1/2
  Constant2/1 -> Switch1/1
  Temperatures1_C/1 -> Bus Creator1/1, Mean/1, Min3/1, Min2/1  "Temperatures_C"
  Temperatures2_C/1 -> Bus Creator2/1, Mean1/1, Min4/1, Min1/1  "Temperatures_C"
  Subtract2/1 -> Bus Creator2/4  "TemperatureDelta_C"
  Min1/1 -> MinimumFunction/3(u2), Add2/1, Bus Creator2/2, Subtract2/2  "T_min"
  Min4/1 -> MaximumFunction/2(u1), Bus Creator2/3, Add2/2, Subtract2/1  "T_max"
  Bus Creator7/1 -> DataPipeline/1  "DataPipeline"
  Bus Creator/1 -> Bus Creator7/2  "VoltageSenseBus"
  Switch/1 -> Bus Creator7/9  "isChargeEn"
  Bus Creator1/1 -> Vector Concatenate/1
  Bus Creator2/1 -> Vector Concatenate/2
  TempSelectForDCL/1 -> Switch4/2
  AverageFunction/1(Average) -> Switch4/1  "AvgTemperature_C"
  Add/1 -> Bus Creator7/4  "DeltaTemperature_C"
  MinimumFunction/1(Min) -> Add/2, Bus Creator7/5  "MinTemperature_C"
  Gain2/1 -> Gain7/1
  Thresholds/1 -> Bus Selector/1  "Thresholds"
  Bus Selector/1 -> GreaterThan/2, Gain/1  "<ChargeDetectionThreshold_mA>"
  ServiceMode/1 -> Bus Creator3/6  "ServiceMode"
  SlowCharge/1 -> Bus Creator3/1  "SlowCharge"
  TransmissionFail/1 -> Bus Creator3/4  "TransmissionFail"
  isChargerConnected/1 -> Bus Creator3/3  "isChargerConnected"
  FastCharge/1 -> Bus Creator3/2  "FastCharge"
  VCUPermanentFail/1 -> Bus Creator3/5  "VCUPermanentFail"
  Gain7/1 -> Bus Creator7/14  "DCL_DisChargingCurrent_A"
  nCellTempGrps/1 -> MinimumFunction/1(n), MaximumFunction/1(n), AverageFunction/3(n)
  SOC/1 -> I2t_perParallelCell/1(SOC), DynamicCurrentLimits_perParallelCell/1(SOC)  "SOC"
  Switch4/1 -> I2t_perParallelCell/2(Temperature_C), DynamicCurrentLimits_perParallelCell/2(Temperature_C)  "Temperature_C"
  DynamicCurrentLimits_perParallelCell/1(DCL_ChargingCurrent_A) -> Gain1/1
  DynamicCurrentLimits_perParallelCell/2(DCL_DisChargingCurrent_A) -> Gain2/1
  Gain1/1 -> Gain6/1
  Mean/1 -> AverageFunction/1(u1)
  Mean1/1 -> AverageFunction/2(u2)
  Vector Concatenate/1 -> Bus Creator7/8  "TemperatureSenseBus"
  isDynamicCurrentEn/1 -> Bus Creator7/10  "isDynamicCurrentEn"
  nCells_Series/1 -> Bus Creator7/11  "nCells_series"
  nCells_Parallel/1 -> Bus Creator7/12  "nCells_parallel"
  Gain3/1 -> Gain4/1
  Gain5/1 -> Gain8/1
  I2t_perParallelCell/2(i2t_Discharge_A2sec) -> Gain5/1
  I2t_perParallelCell/1(i2t_Charge_A2sec) -> Gain3/1
  Gain4/1 -> Bus Creator7/16  "i2t_ChargingCurrent_A2sec"
  Gain8/1 -> Bus Creator7/17  "i2t_DisChargingCurrent_A2sec"
  Bus Creator3/1 -> Bus Selector1/1, Bus Creator7/19  "VCU"
  BalanceEn_atRest/1 -> Bus Creator3/7  "BalanceEn_atRest"
  LoopTimer_SOC_msec/1 -> Bus Creator7/18  "LoopTimer_SOC_msec"
  EmergencyDisconnectEn/1 -> Bus Creator3/8  "EmergencyDisconnectEn"
  Add1/1 -> Bus Creator7/6  "DeltaTemperatureGroup1_C"
  Add2/1 -> Bus Creator7/7  "DeltaTemperatureGroup2_C"
  SlowChargersCurrentLimit_A/1 -> Bus Creator3/9  "SlowChargersCurrentLimit_A"
  MinMax2/1 -> Bus Creator/2, Subtract/2  "mV_min"
  FastChargersCurrentLimit_A/1 -> Bus Creator3/10
  PreChargeLogic/1 -> Bus Creator7/20  "PreChargeLogic"
  MaximumFunction/1(Max) -> Switch4/3, Add/1, Bus Creator7/3  "MaxTemperature_C"
  GetN3/1(NArray) -> MinMax/1, MinMax2/1  "Voltages_mV"
  IR_Calculation_En/1 -> Bus Creator7/22  "IR_Calculation_En"
  TerminalVoltage_mV/1 -> Bus Creator7/21  "TerminalVoltage_mV"
  DynamicCurrentLimits_perParallelCell/3(DCL_arcReactor_A) -> Gain9/1
  Gain10/1 -> Bus Creator7/15  "DCL_arcReactor_A"
  Gain9/1 -> Gain10/1
  IRComplete/1 -> Bus Creator7/26  "IRComplete"
  IRSlowGuard/1 -> Bus Creator7/24  "IRSlowGuard"
  IRFastGuard/1 -> Bus Creator7/25  "IRFastGuard"
  RecordedCycleCount/1 -> Bus Creator7/23  "RecordedCycleCount"
  Bus Selector1/1 -> Display/1  "<SlowCharge>"
  Bus Selector1/2 -> Display1/1  "<FastCharge>"
  Bus Selector1/3 -> Display2/1  "<isChargerConnected>"
  [DCLO_test] -> Bus Creator7/13  "DCL_ChargingCurrent_A"

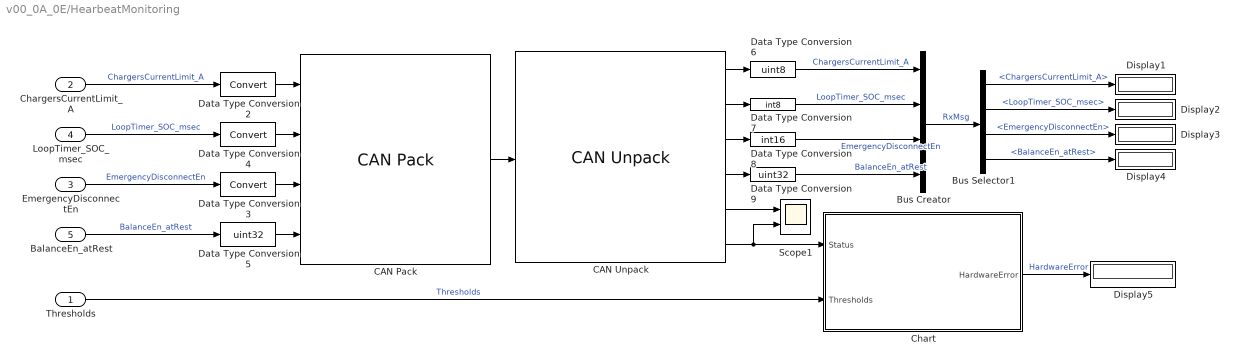
== system v00_0A_0E/HearbeatMonitoring ==
  Thresholds : Inport
  ChargersCurrentLimit_A : Inport  Port=2
  EmergencyDisconnectEn : Inport  Port=3
  LoopTimer_SOC_msec : Inport  Port=4
  BalanceEn_atRest : Inport  Port=5
  Bus Creator : BusCreator  Inputs=4
  Bus Selector1 : BusSelector  OutputSignals=ChargersCurrentLimit_A,LoopTimer_SOC_msec,EmergencyDisconnectEn,BalanceEn_atRest
  CAN Pack : canmsglib/CAN Pack  MsgList=(none)  MsgName=CAN Msg  MsgIDType=Standard (11-bit identifier)  MsgIdentifier=5  MsgLength=8  Remote=off  ApplyMinMax=off  BusOutput=on  SignalInfo={ 'ChargersCurrentLimit_A', '0', '8', 'LE', 'unsigned', 'Standard', '0', '1', '0', '-Inf', 'Inf'; 'LoopTimer_SOC_msec', '8', '8', 'LE', 'signed', 'Standard', '0', '1', '0', '-Inf', 'Inf'; 'EmergencyDisconnectEn', '16', '8', 'LE', 'signed', 'Standard', '0', '1', '0', '-Inf', 'Inf'; 'BalanceEn_atRest', '24', '32', 'LE', 'unsigned', 'Standard', '0', '1', '0', '-Inf', 'Inf' }
      settings: LibrarySourceBlock=embeddedtargetslib/Host Communication/CAN Pack  DataFormat=manually specified signals
  CAN Unpack : canmsglib/CAN Unpack  MsgList=(none)  MsgName=CAN Msg  MsgIDType=Standard (11-bit identifier)  MsgIdentifier=5  MsgLength=8  SignalInfo={ 'ChargersCurrentLimit_A', '0', '8', 'LE', 'unsigned', 'Standard', '0', '1', '0', '-Inf', 'Inf'; 'LoopTimer_SOC_msec', '8', '8', 'LE', 'signed', 'Standard', '0', '1', '0', '-Inf', 'Inf'; 'EmergencyDisconnectEn', '16', '8', 'LE', 'signed', 'Standard', '0', '1', '0', '-Inf', 'Inf'; 'BalanceEn_atRest', '24', '32', 'LE', 'unsigned', 'Standard', '0', '1', '0', '-Inf', 'Inf' }  IDPort=off  TimestampPort=on  ErrorPort=off  RemotePort=off  LengthPort=off  StatusPort=on  ApplyMinMax=off
      settings: LibrarySourceBlock=embeddedtargetslib/Host Communication/CAN Unpack
  Chart : Stateflow chart  TreatAsAtomicUnit=on
  Data Type Conversion2 : DataTypeConversion  SaturateOnIntegerOverflow=off  RndMeth=Floor
  Data Type Conversion3 : DataTypeConversion  SaturateOnIntegerOverflow=off  RndMeth=Floor
  Data Type Conversion4 : DataTypeConversion  SaturateOnIntegerOverflow=off  RndMeth=Floor
  Data Type Conversion5 : DataTypeConversion  OutDataTypeStr=uint32  SaturateOnIntegerOverflow=off  RndMeth=Floor
  Data Type Conversion6 : DataTypeConversion  OutDataTypeStr=uint8  SaturateOnIntegerOverflow=off  RndMeth=Floor
  Data Type Conversion7 : DataTypeConversion  OutDataTypeStr=int8  SaturateOnIntegerOverflow=off  RndMeth=Floor
  Data Type Conversion8 : DataTypeConversion  OutDataTypeStr=int16  SaturateOnIntegerOverflow=off  RndMeth=Floor
  Data Type Conversion9 : DataTypeConversion  OutDataTypeStr=uint32  SaturateOnIntegerOverflow=off  RndMeth=Floor
  Display{1..5} (5 alike) : Display
  Scope1 : Scope  NumInputPorts=2
  wires:
  ChargersCurrentLimit_A/1 -> Data Type Conversion2/1  "ChargersCurrentLimit_A"
  EmergencyDisconnectEn/1 -> Data Type Conversion3/1  "EmergencyDisconnectEn"
  LoopTimer_SOC_msec/1 -> Data Type Conversion4/1  "LoopTimer_SOC_msec"
  BalanceEn_atRest/1 -> Data Type Conversion5/1  "BalanceEn_atRest"
  CAN Pack/1 -> CAN Unpack/1
  Bus Selector1/1 -> Display1/1  "<ChargersCurrentLimit_A>"
  Bus Selector1/2 -> Display2/1  "<LoopTimer_SOC_msec>"
  Bus Selector1/3 -> Display3/1  "<EmergencyDisconnectEn>"
  Bus Selector1/4 -> Display4/1  "<BalanceEn_atRest>"
  Data Type Conversion4/1 -> CAN Pack/2
  Data Type Conversion2/1 -> CAN Pack/1
  Chart/1(HardwareError) -> Display5/1  "HardwareError"
  Data Type Conversion3/1 -> CAN Pack/3
  Data Type Conversion7/1 -> Bus Creator/2  "LoopTimer_SOC_msec"
  Bus Creator/1 -> Bus Selector1/1  "RxMsg"
  CAN Unpack/2 -> Data Type Conversion7/1
  Data Type Conversion9/1 -> Bus Creator/4  "BalanceEn_atRest"
  CAN Unpack/1 -> Data Type Conversion6/1
  CAN Unpack/4 -> Data Type Conversion9/1
  Data Type Conversion8/1 -> Bus Creator/3  "EmergencyDisconnectEn"
  Data Type Conversion6/1 -> Bus Creator/1  "ChargersCurrentLimit_A"
  CAN Unpack/3 -> Data Type Conversion8/1
  Data Type Conversion5/1 -> CAN Pack/4
  Thresholds/1 -> Chart/2(Thresholds)  "Thresholds"
  CAN Unpack/5 -> Scope1/1
  CAN Unpack/6 -> Scope1/2, Chart/1(Status)

== system v00_0A_0E/HearbeatMonitoring_Configuration ==
  Thresholds : Inport
  CAN_Msg : Inport  Port=2
  Bus Creator : BusCreator  Inputs=4
  Bus Selector1 : BusSelector  OutputSignals=ChargersCurrentLimit_A,LoopTimer_SOC_msec,EmergencyDisconnectEn,BalanceEn_atRest
  CAN Unpack : canmsglib/CAN Unpack  MsgList=(none)  MsgName=CAN Msg  MsgIDType=Standard (11-bit identifier)  MsgIdentifier=5  MsgLength=8  SignalInfo={ 'ChargersCurrentLimit_A', '0', '8', 'LE', 'unsigned', 'Standard', '0', '1', '0', '-Inf', 'Inf'; 'LoopTimer_SOC_msec', '8', '16', 'LE', 'signed', 'Standard', '0', '1', '0', '-Inf', 'Inf'; 'EmergencyDisconnectEn', '24', '8', 'LE', 'signed', 'Standard', '0', '1', '0', '-Inf', 'Inf'; 'BalanceEn_atRest', '32', '32', 'LE', 'unsigned', 'Standard', '0', '1', '0', '-Inf', 'Inf' }  IDPort=off  TimestampPort=on  ErrorPort=off  RemotePort=off  LengthPort=off  StatusPort=on  ApplyMinMax=off
      settings: LibrarySourceBlock=embeddedtargetslib/Host Communication/CAN Unpack
  Chart : Stateflow chart  TreatAsAtomicUnit=on
  Data Type Conversion6 : DataTypeConversion  OutDataTypeStr=uint8  SaturateOnIntegerOverflow=off  RndMeth=Floor
  Data Type Conversion7 : DataTypeConversion  OutDataTypeStr=int16  SaturateOnIntegerOverflow=off  RndMeth=Floor
  Data Type Conversion8 : DataTypeConversion  OutDataTypeStr=int16  SaturateOnIntegerOverflow=off  RndMeth=Floor
  Data Type Conversion9 : DataTypeConversion  OutDataTypeStr=uint32  SaturateOnIntegerOverflow=off  RndMeth=Floor
  Display{1..5} (5 alike) : Display
  Scope : Scope  NumInputPorts=4
  Scope1 : Scope  NumInputPorts=2
  wires:
  CAN Unpack/5 -> Scope1/1
  CAN Unpack/6 -> Scope1/2, Chart/1(Status)
  Thresholds/1 -> Chart/2(Thresholds)  "Thresholds"
  CAN Unpack/3 -> Data Type Conversion8/1
  Data Type Conversion6/1 -> Bus Creator/1  "ChargersCurrentLimit_A"
  Data Type Conversion8/1 -> Bus Creator/3  "EmergencyDisconnectEn"
  CAN Unpack/4 -> Data Type Conversion9/1
  CAN Unpack/1 -> Data Type Conversion6/1
  Data Type Conversion9/1 -> Bus Creator/4  "BalanceEn_atRest"
  CAN Unpack/2 -> Data Type Conversion7/1
  Bus Creator/1 -> Bus Selector1/1  "RxMsg"
  Data Type Conversion7/1 -> Bus Creator/2  "LoopTimer_SOC_msec"
  Bus Selector1/4 -> Scope/4, Display4/1  "<BalanceEn_atRest>"
  Bus Selector1/3 -> Display3/1, Scope/3  "<EmergencyDisconnectEn>"
  Bus Selector1/2 -> Display2/1, Scope/2  "<LoopTimer_SOC_msec>"
  Bus Selector1/1 -> Display1/1, Scope/1  "<ChargersCurrentLimit_A>"
  CAN_Msg/1 -> CAN Unpack/1  "CAN Msg"
  Chart/1(HardwareError) -> Display5/1

== system v00_0A_0E/HeartbeatMonitoring_Initial ==
  DataPipeline : Inport
  Bus Selector2 : BusSelector  OutputSignals=VCU.SlowCharge,VCU.isChargerConnected,VCU.EmergencyDisconnectEn,VCU.BalanceEn_atRest
  Chart : Stateflow chart  TreatAsAtomicUnit=on
  Clock : Clock
  Display : Display
  Display1 : Display
  Display2 : Display
  Enabled Subsystem : Subsystem  TreatAsAtomicUnit=on
  IsNaN{,1..3} (4 alike) : RelationalOperator  Operator=isNaN  OutDataTypeStr=boolean  RndMeth=Simplest  InputSameDT=off
  NOR : Logic  Operator=NOR  Inputs=4  IconShape=distinctive  AllPortsSameDT=off  OutDataTypeStr=boolean
  Scope : Scope  NumInputPorts=2
  Signal Builder : Subsystem  Tag=STV Subsys  LoadFcn=sigbuilder_block('load');  StartFcn=sigbuilder_block('start');  StopFcn=sigbuilder_block('stop');  ClipboardFcn=sigbuilder_block('clipboard');  mask(Sigbuilder block){tuvar=[0:10]}
      mask help: Simulink:masks:SigbuilderBlock_MD
      mask init:
      | if ~strcmp(get_param(bdroot(gcbh),'SimulationStatus'),'stopped') tuvar = sigbuilder_block('maskInit'); end
      settings: CopyFcn=sigbuilder_block('copy');  DeleteFcn=sigbuilder_block('delete');  ModelCloseFcn=sigbuilder_block('modelClose');  PreSaveFcn=sigbuilder_block('preSave');  PauseFcn=sigbuilder_block('pause');  ContinueFcn=sigbuilder_block('continue');  NameChangeFcn=sigbuilder_block('namechange');  OpenFcn=sigbuilder_block('open',[0.6 30.6 574.8 555.6 ]);  CloseFcn=sigbuilder_block('close');
      mask Display: plot(0, 0, 100, 100,[2, 2, 32, 32, 2], [68, 8, 8, 68, 68],[32, 2], [38, 38], [32, 19, 2],[53, 60, 44], [32, 17, 17, 2],[16, 16, 31, 31]);txt = getActiveGroup(gcbh);text(2, 100, txt,'verticalAlignment', 'top');
  Terminator : Terminator
  wires:
  DataPipeline/1 -> Bus Selector2/1
  Bus Selector2/2 -> IsNaN1/1  "<isChargerConnected>"
  IsNaN3/1 -> NOR/4
  NOR/1 -> Terminator/1  "VCU_Hearbeat"
  Chart/1(CAN_Transmission) -> Display2/1
  Bus Selector2/4 -> IsNaN3/1  "<BalanceEn_atRest>"
  Bus Selector2/3 -> IsNaN2/1  "<EmergencyDisconnectEn>"
  Bus Selector2/1 -> IsNaN/1  "<SlowCharge>"
  IsNaN2/1 -> NOR/3
  Clock/1 -> Scope/2, Chart/2(ClockTime)
  Signal Builder/1(Signal 1) -> Enabled Subsystem/Enable, Display/1
  Enabled Subsystem/1(Out1) -> Display1/1, Scope/1, Chart/1(HeartbeatCounter)  "HeartbeatCounter"
  IsNaN1/1 -> NOR/2
  IsNaN/1 -> NOR/1

== system v00_0A_0E/HighLevelStatemachine ==
  DataPipeline : Inport
  ContactorCommand : Inport  Port=2
  ContactorsState : Inport  Port=3
  ProtectionOutput : Inport  Port=4
  Thresholds : Inport  Port=5
  HighLevelStatemachine : Stateflow chart  TreatAsAtomicUnit=on
  HighLevelStateMode : Outport
  BMS_State : Outport  Port=2
  wires:
  Thresholds/1 -> HighLevelStatemachine/1(Thresholds)  "Thresholds"
  HighLevelStatemachine/1(HighLevelState) -> HighLevelStateMode/1  "HighLevelStateMode"
  DataPipeline/1 -> HighLevelStatemachine/5(DataPipeline)  "DataPipeline"
  ProtectionOutput/1 -> HighLevelStatemachine/4(ProtectionOutput)  "ProtectionOutput"
  ContactorsState/1 -> HighLevelStatemachine/3(ContactorsState)
  HighLevelStatemachine/2(BMS_State) -> BMS_State/1  "BMS_State"
  ContactorCommand/1 -> HighLevelStatemachine/2(ContactorCommand)

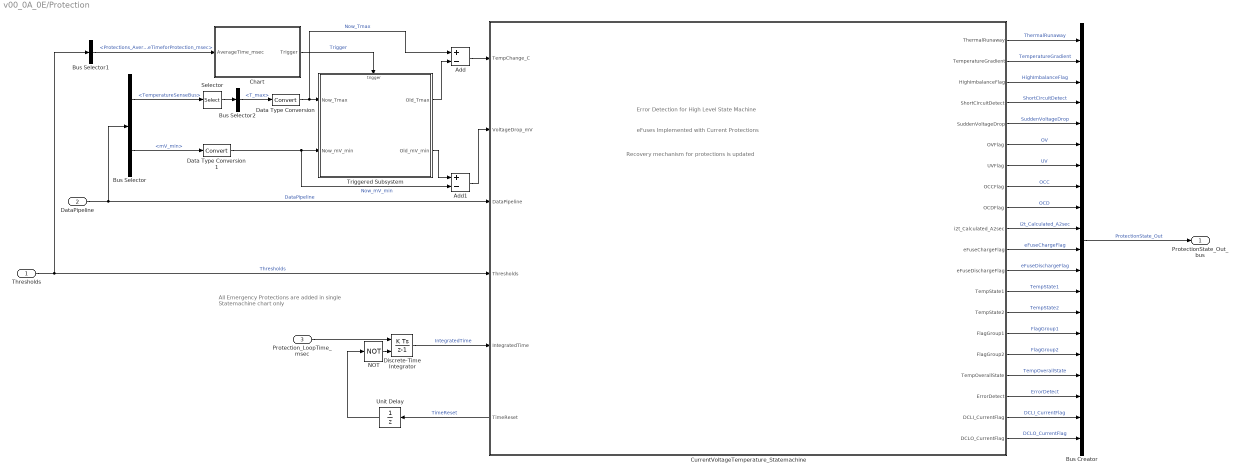
== system v00_0A_0E/Protection ==
  note: eFuses Implemented with Current Protections
  note: All Emergency Protections are added in single Statemachine chart only
  note: Recovery mechanism for protections is updated
  note: Error Detection for High Level State Machine
  Thresholds : Inport
  DataPipeline : Inport  Port=2
  Protection_LoopTime_msec : Inport  Port=3
  Add : Sum  Inputs=+-
  Add1 : Sum  Inputs=+-
  Bus Creator : BusCreator  Inputs=20  OutDataTypeStr=Bus: ProtectionState_Out  NonVirtualBus=on
  Bus Selector : BusSelector  OutputSignals=TemperatureSenseBus,VoltageSenseBus.mV_min
  Bus Selector1 : BusSelector  OutputSignals=Protections_AverageTimeforProtection_msec
  Bus Selector2 : BusSelector  OutputSignals=T_max
  Chart : Stateflow chart  TreatAsAtomicUnit=on
  CurrentVoltageTemperature_Statemachine : Stateflow chart  TreatAsAtomicUnit=on
      settings: PortSchema="{\"entries\":[{\"content\":{\"sides\":[{\"content\":{\"connectorIds\":[\"In1\",\"In2\",\"In4\",\"In3\",\"In5\",\"Out21\"]},\"type\":\"ConnectorPlacement.EquallySpacedRectSide\",\"uuid\":\"96c9cb3b-ce9e-40bc-83f0-1b33c5331fb0\"},{\"content\":{\"connectorIds\":[\"Out9\",\"Out10\",\"Out11\",\"Out12\",\"Out13\",\"Out3\",\"Out4\",\"Out1\",\"Out2\",\"Out16\",\"Out18\",\"Out17\",\"Out6\",\"Out5\",\"Out7\",\"Out8\",\"Out15\",\"Out14\",\"Out19\",\"Out20\"],\"side\":\"RIGHT\"},\"type\":\"ConnectorPlacement.EquallySpacedRectSide\",\"uuid\":\"ee7657d7-c960-4f1a-8166-b0da65e70191\"},{\"content\":{\"connectorIds\":[],\"side\":\"TOP\"},\"type\":\"ConnectorPlacement.EquallySpacedRectSide\",\"uuid\":\"5531a0de-ea25-43be-85f9-34afd340e6a9\"}]},\"type\":\"ConnectorPlacement.EquallySpacedConnector\",\"uuid\":\"8d856e57-f114-48c3-9d7e-532a4ebae39d\"}],\"packageUris\":[\"http://schema.mathworks.com/mf0/Connector/R2020b\"],\"version\":\"1.0\"}"
  Data Type Conversion : DataTypeConversion  SaturateOnIntegerOverflow=off  RndMeth=Floor
  Data Type Conversion1 : DataTypeConversion  SaturateOnIntegerOverflow=off  RndMeth=Floor
  Discrete-Time Integrator : DiscreteIntegrator  gainval=1  ExternalReset=level  SampleTime=-1  ICPrevOutput=DiscIntNeverNeededParam  ICPrevScaledInput=DiscIntNeverNeededParam
  NOT : Logic  Operator=NOT  IconShape=distinctive  AllPortsSameDT=off  OutDataTypeStr=boolean
  Selector : Selector  InputPortWidth=2  IndexOptions=Index vector (dialog)  Indices=[1]  OutputSizes=1
  Triggered Subsystem : Subsystem  TreatAsAtomicUnit=on
  Unit Delay : UnitDelay  SampleTime=-1  HasFrameUpgradeWarning=on
  ProtectionState_Out_bus : Outport
  wires:
  Bus Creator/1 -> ProtectionState_Out_bus/1  "ProtectionState_Out"
  Thresholds/1 -> Bus Selector1/1, CurrentVoltageTemperature_Statemachine/3(Thresholds)  "Thresholds"
  Bus Selector/2 -> Data Type Conversion1/1  "<mV_min>"
  DataPipeline/1 -> Bus Selector/1, CurrentVoltageTemperature_Statemachine/4(DataPipeline)  "DataPipeline"
  CurrentVoltageTemperature_Statemachine/9(ThermalRunaway) -> Bus Creator/1  "ThermalRunaway"
  CurrentVoltageTemperature_Statemachine/10(TemperatureGradient) -> Bus Creator/2  "TemperatureGradient"
  CurrentVoltageTemperature_Statemachine/11(HighImbalanceFlag) -> Bus Creator/3  "HighImbalanceFlag"
  CurrentVoltageTemperature_Statemachine/12(ShortCircuitDetect) -> Bus Creator/4  "ShortCircuitDetect"
  CurrentVoltageTemperature_Statemachine/13(SuddenVoltageDrop) -> Bus Creator/5  "SuddenVoltageDrop"
  CurrentVoltageTemperature_Statemachine/3(OVFlag) -> Bus Creator/6  "OV"
  CurrentVoltageTemperature_Statemachine/4(UVFlag) -> Bus Creator/7  "UV"
  CurrentVoltageTemperature_Statemachine/1(OCCFlag) -> Bus Creator/8  "OCC"
  CurrentVoltageTemperature_Statemachine/2(OCDFlag) -> Bus Creator/9  "OCD"
  CurrentVoltageTemperature_Statemachine/16(i2t_Calculated_A2sec) -> Bus Creator/10  "i2t_Calculated_A2sec"
  CurrentVoltageTemperature_Statemachine/18(eFuseChargeFlag) -> Bus Creator/11  "eFuseChargeFlag"
  CurrentVoltageTemperature_Statemachine/17(eFuseDischargeFlag) -> Bus Creator/12  "eFuseDischargeFlag"
  CurrentVoltageTemperature_Statemachine/6(TempState1) -> Bus Creator/13  "TempState1"
  CurrentVoltageTemperature_Statemachine/5(TempState2) -> Bus Creator/14  "TempState2"
  CurrentVoltageTemperature_Statemachine/7(FlagGroup1) -> Bus Creator/15  "FlagGroup1"
  CurrentVoltageTemperature_Statemachine/8(FlagGroup2) -> Bus Creator/16  "FlagGroup2"
  CurrentVoltageTemperature_Statemachine/15(TempOverallState) -> Bus Creator/17  "TempOverallState"
  CurrentVoltageTemperature_Statemachine/14(ErrorDetect) -> Bus Creator/18  "ErrorDetect"
  Selector/1 -> Bus Selector2/1
  Bus Selector/1 -> Selector/1  "<TemperatureSenseBus>"
  Bus Selector2/1 -> Data Type Conversion/1  "<T_max>"
  Data Type Conversion/1 -> Add/1, Triggered Subsystem/1(Now_Tmax)  "Now_Tmax"
  Chart/1(Trigger) -> Triggered Subsystem/Trigger  "Trigger"
  Data Type Conversion1/1 -> Add1/2, Triggered Subsystem/2(Now_mV_min)  "Now_mV_min"
  Bus Selector1/1 -> Chart/1(AverageTime_msec)  "<Protections_AverageTimeforProtection_msec>"
  Triggered Subsystem/1(Old_Tmax) -> Add/2
  Triggered Subsystem/2(Old_mV_min) -> Add1/1
  Add1/1 -> CurrentVoltageTemperature_Statemachine/2(VoltageDrop_mV)
  Add/1 -> CurrentVoltageTemperature_Statemachine/1(TempChange_C)
  CurrentVoltageTemperature_Statemachine/19(DCLI_CurrentFlag) -> Bus Creator/19  "DCLI_CurrentFlag"
  CurrentVoltageTemperature_Statemachine/20(DCLO_CurrentFlag) -> Bus Creator/20  "DCLO_CurrentFlag"
  CurrentVoltageTemperature_Statemachine/21(TimeReset) -> Unit Delay/1  "TimeReset"
  Discrete-Time Integrator/1 -> CurrentVoltageTemperature_Statemachine/5(IntegratedTime)  "IntegratedTime"
  Protection_LoopTime_msec/1 -> Discrete-Time Integrator/1
  Unit Delay/1 -> NOT/1
  NOT/1 -> Discrete-Time Integrator/2
